simulink library "Lib_JARVISPH2_deVCU_Com"  (R2019b)
settings: Solver=ode45  StartTime=0.0  StopTime=10.0  RelTol=1e-3  EnableMultiTasking=on
settings Model: Creator=kmansour  LastModifiedBy=User
settings DataIOCC: LimitDataPoints=on  SaveFormat=Array  ReturnWorkspaceOutputs=off
settings OptimizationCC: LifeSpan=inf
settings DebuggingCC: AllowSymbolicDim=off  SFUnexpectedBacktrackingDiag=warning  SFNoUnconditionalDefaultTransitionDiag=warning  SFExecutionAtInitializationDiag=none  ArithmeticOperatorsInVariantConditions=warning
settings HardwareCC: ProdBitPerPointer=32  ProdBitPerSizeT=32  ProdBitPerPtrDiffT=32  ProdLargestAtomicFloat=None  ProdIntDivRoundTo=Undefined  ProdEndianess=Unspecified  ProdWordSize=32  ProdHWDeviceType=32-bit Generic
settings ModelReferenceCC: PropagateSignalLabelsOutOfModel=off
settings SFSimCC: SimUseLocalCustomCode=off  CustomCodeUndefinedFunction=UseInterfaceOnly
settings RTWCC: RTWUseLocalCustomCode=off
settings CodeAppCC: StateflowObjectComments=on
settings GRTTargetCC: TargetLangStandard=C89/C90 (ANSI)  GeneratePreprocessorConditionals=Disable all
settings ConfigComp: CovMetricSettings=dw  CovHtmlReporting=on  CovSaveCumulativeToWorkspaceVar=on  CovSaveSingleToWorkspaceVar=on  CovExternalEMLEnable=off

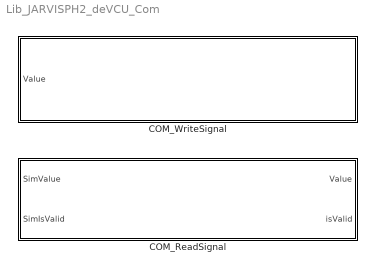
== system Lib_JARVISPH2_deVCU_Com ==
  COM_ReadSignal : Subsystem  TreatAsAtomicUnit=on  mask{PARAM_ID=APP_RX_ABS_EBS_AMBER_WARNING_LAMP_STATE}
      mask prompts: PARAM_ID "Choose Signal"
      mask TypeOptions PARAM_ID: APP_RX_ABS_EBS_AMBER_WARNING_LAMP_STATE | APP_RX_ABS_FULLY_OPERATIONAL | APP_RX_ABS_OFFROAD_SWITCH | APP_RX_ACCPEDAL_POS1 | APP_RX_ACC_PEDAL1LOWIDLESWITCH | APP_RX_ACC_PEDAL2KICKDOWNSWITCH | APP_RX_ACC_PEDAL_FAULT_BYTE1 | APP_RX_ACC_PEDAL_FAULT_BYTE2 | APP_RX_ACC_PEDAL_FAULT_BYTE3 | APP_RX_ACC_PEDAL_FAULT_BYTE4 | APP_RX_ACC_PEDAL_FAULT_BYTE5 | APP_RX_ACC_PEDAL_FAULT_BYTE6 | APP_RX_ACC_PEDAL_FAULT_BYTE7 | APP_RX_ACC_PEDAL_FAULT_BYTE8 | APP_RX_ACLTR_INTERLOCK_SWITCH | APP_RX_ACTUAL_TEMP_PUMP_AIRCOMP | APP_RX_AIR_COMPRESSOR_STATUS | APP_RX_AIR_SUSPENSION_SUPPLY_PRESSURE | APP_RX_AMBIENTTEMPERATURE | APP_RX_ANTI_LOCK_BRAKING_ABS_ACTIVE | APP_RX_ASR_BRAKE_CTRL_ACTIVE | APP_RX_ASR_ENG_CTRL_ACTIVE | APP_RX_ASR_HILL_HOLDER_SWITCH | APP_RX_ASR_OFFROAD_SWITCH | APP_RX_ATC_ASR_INFORMATION_SIGNAL | APP_RX_AUXILIARYVOLTAGE | APP_RX_AUXILIARYVOLTAGESTATUS | APP_RX_AUXILIARY_EQUIPMENT_SUPPLY_PRESS | APP_RX_BATTERY_SOH | APP_RX_BMS_CHECKSUM_126 | APP_RX_BMS_DCBUSVOLTAGE | APP_RX_BMS_HIGHESTINLETTEMP | APP_RX_BMS_HIGHESTOUTLETTEMP | APP_RX_BMS_MAXBATVOLTALLOWED | APP_RX_BMS_MAXCELLTEMP | APP_RX_BMS_MAXCONTCHRGCURRENT | APP_RX_BMS_MAXCONTDISCHRGCURRENT | APP_RX_BMS_MESSAGECOUNTER_126_HEARTBEAT | APP_RX_BMS_MINCELLTEMP | APP_RX_BMS_PACKCURRENT | APP_RX_BMS_PACKSTATE | APP_RX_BMS_PACKVOLTAGE | APP_RX_BMS_SOC | APP_RX_BMS_SUBPACK10STATUS | APP_RX_BMS_SUBPACK11STATUS | APP_RX_BMS_SUBPACK12STATUS | APP_RX_BMS_SUBPACK13STATUS | APP_RX_BMS_SUBPACK14STATUS | APP_RX_BMS_SUBPACK15STATUS | APP_RX_BMS_SUBPACK16STATUS | APP_RX_BMS_SUBPACK1STATUS | APP_RX_BMS_SUBPACK2STATUS | APP_RX_BMS_SUBPACK3STATUS | APP_RX_BMS_SUBPACK4STATUS | APP_RX_BMS_SUBPACK5STATUS | APP_RX_BMS_SUBPACK6STATUS | APP_RX_BMS_SUBPACK7STATUS | APP_RX_BMS_SUBPACK8STATUS | APP_RX_BMS_SUBPACK9STATUS | APP_RX_BMS_SYSTEMISORES | APP_RX_BMS_TMAX_CELL_ID | APP_RX_BMS_TMAX_SUBPACK_ID | APP_RX_BMS_TMIN_CELL_ID | APP_RX_BMS_TMIN_SUBPACK_ID | APP_RX_BRAKE_PEDAL_POSITION | APP_RX_CHECKSUM_122 | APP_RX_CHECKSUM_123 | APP_RX_COMMANDMODE_MCUCMD1RES | APP_RX_CONNECTED_STRING | APP_RX_DC_LINK_VOLTAGE_VCU_RX | APP_RX_DETECTED_STRING | APP_RX_EBS_BRAKE_SWITCH | APP_RX_EBS_RED_WARNING_LAMP_STATE | APP_RX_EM1_MESSAGECHECKSUM | APP_RX_EM1_MESSAGECOUNTER | APP_RX_EM1_OVR_CTRL_MODE_BRAKING | APP_RX_EM1_OVR_CTRL_MODE_DRIVING | APP_RX_EM1_OVR_CTRL_MODE_PRIO_BRAKING | APP_RX_EM1_OVR_CTRL_MODE_PRIO_DRIVING | APP_RX_EM1_REQ_TRQ_TRQ_LIMIT_BRAKING | APP_RX_EM1_REQ_TRQ_TRQ_LIMIT_DRIVING | APP_RX_EMERGENCYSTOP | APP_RX_EMITEMPERATURE | APP_RX_ENG_RET_SELECTION | APP_RX_EVENTID | APP_RX_FAULTDRIVECOVERWASOPENED | APP_RX_FAULTDRIVECOVERWASOPENEDSTATUS | APP_RX_FAULTINTERLOCKBATTERYCABLE | APP_RX_FAULTINTERLOCKBATTERYCABLESTATUS | APP_RX_FAULTINTERLOCKMOTORCABLE | APP_RX_FAULTINTERLOCKMOTORCABLESTATUS | APP_RX_FAULTPHASETOCHASSIS | APP_RX_FAULTPHASETOCHASSISSTATUS | APP_RX_FAULT_CODE_EHVS_VCU_RX | APP_RX_G1CHARGER_GUN_DETECTED | APP_RX_G1CHARGING_STATUS | APP_RX_G1DIFF_CURRENT_MEASURE | APP_RX_G1EVCC_READY | APP_RX_G1EVCC_STATUS_CODE | APP_RX_G1GUN_LOCK_FAULT | APP_RX_G1NEGATIVE_CONTACTOR_CONTROL | APP_RX_G1POSITIVE_CONTACTOR_CONTROL | APP_RX_G1TEMPERATURE1_FAULT | APP_RX_G1TEMPERATURE2_FAULT | APP_RX_G1TEMPERATURE_1_VAL | APP_RX_G1TEMPERATURE_2_VAL | APP_RX_G1VEHICLE_IMMOBILIZE | APP_RX_G1_GUNLOCKFEEDBACK | APP_RX_G2CHARGER_GUN_DETECTED | APP_RX_G2CHARGING_STATUS | APP_RX_G2DIFF_CURRENT_MEASURE | APP_RX_G2EVCC_READY | APP_RX_G2EVCC_STATUS_CODE | APP_RX_G2GUN_LOCK_FAULT | APP_RX_G2NEGATIVE_CONTACTOR_CONTROL | APP_RX_G2POSITIVE_CONTACTOR_CONTROL | APP_RX_G2TEMPERATURE1_FAULT | APP_RX_G2TEMPERATURE2_FAULT | APP_RX_G2TEMPERATURE_1_VAL | APP_RX_G2TEMPERATURE_2_VAL | APP_RX_G2VEHICLE_IMMOBILIZE | APP_RX_G2_GUNLOCKFEEDBACK | APP_RX_GEARSELECTOR_TESTSIG1 | APP_RX_GEARSELECTOR_TESTSIG2 | APP_RX_HALT_BRAKE_SWITCH | APP_RX_HIGHPOWERCURRENT | APP_RX_HIGHPOWERCURRENTSTATUS | APP_RX_HIGHPOWERVOLTAGE | APP_RX_HIGHPOWERVOLTAGESTATUS | APP_RX_HV_CONTACTOR_STATUS | APP_RX_MAXSAFEMOTORSPEEDFORWARD | APP_RX_MAXSAFEMOTORSPEEDFORWARDSTATUS | APP_RX_MAXSAFEMOTORSPEEDREVERSE | APP_RX_MAXSAFEMOTORSPEEDREVERSESTATUS | APP_RX_MCUPOLLINGVMU_BYTE1 | APP_RX_MCUPOLLINGVMU_BYTE2 | APP_RX_MCUPOLLINGVMU_BYTE3 | APP_RX_MCUPOLLINGVMU_BYTE4 | APP_RX_MCUPOLLINGVMU_BYTE5 | APP_RX_MCUPOLLINGVMU_BYTE6 | APP_RX_MCUPOLLINGVMU_BYTE7 | APP_RX_MCUPOLLINGVMU_BYTE8 | APP_RX_MCUTEMPERATURE | APP_RX_MCU_POLLING_MCU_BYTE1 | APP_RX_MCU_POLLING_MCU_BYTE2 | APP_RX_MCU_POLLING_MCU_BYTE3 | APP_RX_MCU_POLLING_MCU_BYTE4 | APP_RX_MCU_POLLING_MCU_BYTE5 | APP_RX_MCU_POLLING_MCU_BYTE6 | APP_RX_MCU_POLLING_MCU_BYTE7 | APP_RX_MCU_POLLING_MCU_BYTE8 | APP_RX_MESSAGECOUNTER_122 | APP_RX_MOTORANGLE | APP_RX_MOTORANGLESTATUS | APP_RX_MOTORSPEED | APP_RX_MOTORSPEEDSTATUS | APP_RX_MOTORTEMPERATURE | APP_RX_MOTORTORQUEESTIMATED | APP_RX_MOTORTORQUEESTIMATEDSTATUS | APP_RX_OPERATIONALMODE_MCUCMD1RES | APP_RX_OUTPUT_CURRENT_AIRCOMP | APP_RX_OUTPUT_CURRENT_EHVS | APP_RX_PARKING_AND_OR_TRAILER_AIR_PRESS | APP_RX_PNEUMATIC_SUPPLY_PRESSURE | APP_RX_PUMPCOMMUNICATIONFAULT | APP_RX_PUMPCURRENT | APP_RX_PUMPDRYRUNFAULT | APP_RX_PUMPFAULTLEVEL | APP_RX_PUMPOVERCURRENTFAULT | APP_RX_PUMPOVERVOLTAGEFAULT | APP_RX_PUMPSPEED | APP_RX_PUMPSTALLFAULT | APP_RX_PUMPTEMP | APP_RX_PUMPTHERMALFAULT | APP_RX_PUMPUNDERVOLTAGEFAULT | APP_RX_PUMPVOLTAGE | APP_RX_REGENDERATING | APP_RX_REGENDERATINGSTATUS | APP_RX_REGENTORQUEAVAIL | APP_RX_REGENTORQUEAVAILSTATUS | APP_RX_ROLLINGCOUNTER_MCUCMD1RESPONSE | APP_RX_ROLLINGCOUNTER_MCUCMD2RESPONSE | APP_RX_ROLLINGCOUNTER_MCUINFO1 | APP_RX_ROLLINGCOUNTER_MCUINFO2 | APP_RX_ROLLINGCOUNTER_MCUONEVENTINFO1 | APP_RX_ROLLINGCOUNTER_MCUTHERMAL2 | APP_RX_SA_OF_CTRLLINGDEVICEFORBRAKECTRL | APP_RX_SERVICE_BRAKE_CIRCUIT_1_AIR_PRES | APP_RX_SERVICE_BRAKE_CIRCUIT_2_AIR_PRES | APP_RX_SPEEDREDUCTIONREQUEST | APP_RX_STATEMCU | APP_RX_STATUSU0_FAULT_EHVS_VCU_RX | APP_RX_STATUSU0_OVERCURRENTFAULT_EHVS_V | APP_RX_STATUSU0_WARNING_EHVS_VCU_RX | APP_RX_STATUSU1_FAULT_AIRCOMP_VCU_RX | APP_RX_STATUSU1_OVERCURRENT_AIRCOMP_VCU | APP_RX_STATUSU1_OVERTEMP_AIRCOMP_VCU_RX | APP_RX_STATUSU1_WARNING_AIRCOMP_VCU_RX | APP_RX_SWITCHING_SYNC_STATUS | APP_RX_SYS_DTC | APP_RX_T2B_BMS_WORK_MODE | APP_RX_T2B_COMP_FREQUENCY | APP_RX_T2B_COOLANT_IN_TEMP | APP_RX_T2B_COOLANT_OUT_TEMP | APP_RX_T2B_FAULT_CODE | APP_RX_T2B_MODE | APP_RX_T2B_SIGNAL_LIFE | APP_RX_T2B_TMS_WORK_MODE | APP_RX_TRACTIONDERATING | APP_RX_TRACTIONDERATINGSTATUS | APP_RX_TRACTIONTORQUEAVAIL | APP_RX_TRACTIONTORQUEAVAILSTATUS | APP_RX_TRACTION_CTRL_OVR_SWITCH | APP_RX_TRAILER_ABS_STATUS | APP_RX_TRAILER_ABS_WARNING_SIGNAL | APP_RX_TRANSREQUEST_GEAR
      mask Display:
      | image(imread('devcu_final.png'),'top-left');
      | color('black');
      | port_label('input', 1, 'SimValue');
      | port_label('input', 2, 'SimIsValid');
      | port_label('output', 1, 'Value');
      | port_label('output', 2, 'isValid');
      | 
      | strCell =get_param(gcb, 'MaskValues');
      | strCell = strtrim(strCell);
      | str = strCell{1};
      | str = strrep(str, '_', '\_');
      | disp(str, 'texmode', 'on');
  COM_WriteSignal : Subsystem  TreatAsAtomicUnit=on  mask{PARAM_ID=APP_TX_ACKNOWLEDGEMENT}
      mask prompts: PARAM_ID "Choose Signal"
      mask TypeOptions PARAM_ID: APP_TX_ACKNOWLEDGEMENT | APP_TX_AIR_COMPRESSOR_AVAILABLE | APP_TX_AMBER_WARNING_LAMP_CHECK_HV | APP_TX_AP_LOW_IDLE_SWITCH | APP_TX_B2T_BATTERY_AVG_TEMP | APP_TX_B2T_BMS_WORK_MODE | APP_TX_B2T_COMP_SPEED_RESTRICTION | APP_TX_B2T_DIFFERENTIAL1 | APP_TX_B2T_DIFFERENTIAL2 | APP_TX_B2T_MODE | APP_TX_B2T_SET_TARGET_TEMP | APP_TX_B2T_SIGNAL_LIFE | APP_TX_B2T_TCELL_MAX | APP_TX_B2T_TCELL_MIN | APP_TX_B2T_TMS_CONTROL_CMD | APP_TX_BOOTNUMBER | APP_TX_CHECKSUM_200 | APP_TX_COMMANDMODEEXT | APP_TX_COMMANDMODE_VMUCMD2 | APP_TX_CONTROL0_EHPS | APP_TX_CONTROL1_AIRCOMP | APP_TX_DCDCONOFF | APP_TX_DISTANCE_TO_EMPTY_DTE | APP_TX_DTC_ACCHALLSENSOR_MALF_EXT_ERROR | APP_TX_DTC_ACCPDL_CHECKSUM_ERROR | APP_TX_DTC_ACCPDL_OUT_OF_CALIBRATION | APP_TX_DTC_ACCPDL_OVERTRAVEL_CLOCKWISE | APP_TX_DTC_ACCPDL_OVERTRAVEL_CNTRCW | APP_TX_DTC_ACC_HALLSENS_MALF_INT_ERROR | APP_TX_DTC_AIRCOMP_WARNING | APP_TX_DTC_AIR_COMPRESSOR_FAULT_ACTIVE | APP_TX_DTC_AIR_COMP_NOT_FUNCTIONAL | APP_TX_DTC_AUXBATT_UV_ACTIVE_WARN | APP_TX_DTC_AUX_BATTERY_OVER_VOLTAGE | APP_TX_DTC_AUX_BATTERY_UNDER_VOLTAGE | APP_TX_DTC_BATTERY_PACK_EMPTY_LOW_SOC | APP_TX_DTC_BATTTEMPLIMREACHEDDRNGCHRG | APP_TX_DTC_BATT_INTERNALLYWELDEDCONT | APP_TX_DTC_BRAKE_AIRCOMP_OVERCURRENT | APP_TX_DTC_BRAKE_AIRCOMP_OVERHEAT | APP_TX_DTC_CHARGE_COMPLETE | APP_TX_DTC_CHARSYSTEM_NOT_COMPATIBLE | APP_TX_DTC_DC_LINK_VOLTAGE_NOT_NORMAL | APP_TX_DTC_EHPS_FAULT_ACTIVE | APP_TX_DTC_EHPS_NOT_FUNCTIONAL | APP_TX_DTC_EHPS_OVERCURRENT | APP_TX_DTC_EHPS_WARNING | APP_TX_DTC_GUN1CHRG_CABLE_CHECK_FAILED | APP_TX_DTC_GUN1_CHARGING_AUTH_FAILED | APP_TX_DTC_GUN1_CHARGING_INIT_FAILED | APP_TX_DTC_GUN1_CONTACTORS_WELDED | APP_TX_DTC_GUN1_CONTACTOR_OPERFAULT | APP_TX_DTC_GUN1_LOCK_FAULT | APP_TX_DTC_GUN1_PRECHARGE_FAILED | APP_TX_DTC_GUN1_STOP_CHARGING_FLAG | APP_TX_DTC_GUN2_CHARGING_AUTH_FAILED | APP_TX_DTC_GUN2_CHARGING_INIT_FAILED | APP_TX_DTC_GUN2_CHRGCABLE_CHECK_FAILED | APP_TX_DTC_GUN2_CONTACTORS_WELDED | APP_TX_DTC_GUN2_CONT_OPERATION_FAULT | APP_TX_DTC_GUN2_LOCK_FAULT | APP_TX_DTC_GUN2_PRECHARGE_FAILED | APP_TX_DTC_GUN2_STOP_CHARGING_FLAG | APP_TX_DTC_HVAC_AMBIENT_SENSOR_FAULT | APP_TX_DTC_HVAC_CABIN_SENSOR_FAULT | APP_TX_DTC_HVAC_CAN_COMM_FAULT | APP_TX_DTC_HVAC_COMPRESSOR_FAULT | APP_TX_DTC_HVAC_COOLANT_LOW | APP_TX_DTC_HVAC_COOLANT_OVERHEAT | APP_TX_DTC_HVAC_DCDC_FAULT | APP_TX_DTC_HVAC_PRESSURE_FAULT | APP_TX_DTC_HVAC_PUMP_COMM_ERROR | APP_TX_DTC_HVAC_PUMP_DRY_RUN_FAULT | APP_TX_DTC_HVAC_PUMP_OVERCURRENT | APP_TX_DTC_HVAC_PUMP_OVERHEAT | APP_TX_DTC_HVAC_PUMP_STALL_FAULT | APP_TX_DTC_HVAC_SUCTION_TEMPSEN_FAULT | APP_TX_DTC_HVAC_WATERIN_SENSOR_FAULT | APP_TX_DTC_HVAC_WATEROUT_SENSOR_FAULT | APP_TX_DTC_HVIL_JB | APP_TX_DTC_IMBALANCED_STRING | APP_TX_DTC_IRREGULAR_INPUT_FROM_USER | APP_TX_DTC_KEY_NOT_DETECTED | APP_TX_DTC_LID_OPEN | APP_TX_DTC_LOSTCOMWITHMODULEINASTRING | APP_TX_DTC_LOST_COMM_WITH_HOST | APP_TX_DTC_LOST_COMM_WITH_SLAVES | APP_TX_DTC_MALFUNC_ACCPEDAL_WHILE_RUN | APP_TX_DTC_MANIPULATED_ACCPEDAL_VALUES | APP_TX_DTC_MCU_COMM_TIMEOUT_ERROR | APP_TX_DTC_MCU_EMERGENCY_STOP_REQUESTED | APP_TX_DTC_MCU_FAILED_TO_INITIALIZE | APP_TX_DTC_MCU_FAILURE | APP_TX_DTC_MCU_FAILUREDUETOOVERTEMP | APP_TX_DTC_MCU_FAULT_OBSERVED | APP_TX_DTC_MCU_OPERATIONAL_FAULT | APP_TX_DTC_MCU_OVERTEMP_WARNING | APP_TX_DTC_MCU_TEMP_LIMIT_REACHED | APP_TX_DTC_MOTOR_OVERTEMP_WARNING | APP_TX_DTC_MOTOR_TEMP_LIMIT_REACHED | APP_TX_DTC_PDU_CONTACTOR_WELDED | APP_TX_DTC_PDU_CONT_OPER_FAULT | APP_TX_DTC_PRECHARGE_FAULT | APP_TX_DTC_REFUSED_ENTER_NEUTRAL_MODE | APP_TX_DTC_REFUSED_ENTER_REVERSE_MODE | APP_TX_DTC_REFUSED_TO_ENTER_DRIVE_MODE | APP_TX_DTC_RISO_FAULT | APP_TX_DTC_SW_NOT_INSTALLED_PROPERLY | APP_TX_DTC_SYSTEM_CURRENT_CONTROL_FAULT | APP_TX_DTC_SYSTEM_LEVEL_BATTERY_FAULT | APP_TX_DTC_TCSCOOLANTINTEMPSENSOR_FAULT | APP_TX_DTC_TCSCOOLANTOUTTEMPSENS_FAULT | APP_TX_DTC_TCS_COOLANT_LEVEL_LOW | APP_TX_DTC_TCS_COOLANT_OUTLET_TEMP_HIGH | APP_TX_DTC_TCS_COOLANT_OVERHEAT | APP_TX_DTC_TCS_PUMP_COMM_FAULT | APP_TX_DTC_TCS_PUMP_OVERCURRENT_FAULT | APP_TX_DTC_TCS_PUMP_STALL_FAULT | APP_TX_DTC_TCS_PUMP_THERMAL_FAULT | APP_TX_DTC_TRQ_LIM_DUE_TO_MCU_DERATING | APP_TX_DTC_TRQ_LIM_DUE_TO_OVERCURRENT | APP_TX_DTC_TRQ_LIM_DUE_TO_OVERSPEED | APP_TX_DTC_TRQ_LIM_DUE_TO_THERMAL_LIM | APP_TX_DTC_TRQ_LIM_MCU_OUTOFORDER | APP_TX_DTC_VEHICLESYSTEM_NOT_COMPATIBLE | APP_TX_DTC_VEHICLE_CAN1_BUS_INACTIVE | APP_TX_DTC_VEHICLE_CAN2_BUS_INACTIVE | APP_TX_DTC_VEHICLE_CAN3_BUS_INACTIVE | APP_TX_EM1_ACTUAL_MAXAVAILRETPCTTRQ | APP_TX_EM1_ACTUAL_PCT_TORQUE | APP_TX_EM1_DRIVER_RETARDER_PCT_TORQUE | APP_TX_EM1_EMOTOR_OUTPUT_SHAFT_SPEED | APP_TX_EM1_ER_SEQUENCE_NUMBER | APP_TX_EM1_REF_ENG_TORQ | APP_TX_EM1_REF_RET_TORQ | APP_TX_EM1_RET_LOCATION | APP_TX_EM1_RET_SELECTION_NON_ENG | APP_TX_EM1_RET_TYPE | APP_TX_EM1_SA_OF_CTRL_DEVICE | APP_TX_EM1_TORQUE_MODE_DRIVING_BRAKING | APP_TX_G1BATTERY_PACK_PRESENT_VOLT | APP_TX_G1CHARG_COMP_FLAG | APP_TX_G1EV_CONTI_CHARG_CUR_LIMIT | APP_TX_G1EV_ERROR_CODE | APP_TX_G1EV_MAX_CHARG_CUR_LIMIT | APP_TX_G1EV_READY_FLAG | APP_TX_G1NOMI_BATT_CAPA | APP_TX_G1REMAIN_BATT_CAPA | APP_TX_G1SOC | APP_TX_G1VEHI_STOP_CHARG_FLAG | APP_TX_G2BATTERY_PACK_PRESENT_VOLT | APP_TX_G2CHARG_COMP_FLAG | APP_TX_G2EV_CONTI_CHARG_CUR_LIMIT | APP_TX_G2EV_ERROR_CODE | APP_TX_G2EV_MAX_CHARG_CUR_LIMIT | APP_TX_G2EV_READY_FLAG | APP_TX_G2NOMI_BATT_CAPA | APP_TX_G2REMAIN_BATT_CAPA | APP_TX_G2SOC | APP_TX_G2VEHI_STOP_CHARG_FLAG | APP_TX_HIGH_VOLT_BATT_1_FAULT | APP_TX_HIGH_VOLT_BATT_2_FAULT | APP_TX_HOST_BMSSTATEREQUEST | APP_TX_HV_READY | APP_TX_HV_SYSTEM_VOLTAGE | APP_TX_INVERTER_TEMPERATURE | APP_TX_MAJORMCUPROTOCOL | APP_TX_MAXBATTERYVOLTAGE | APP_TX_MAXBATTERYVOLTAGESTATUS | APP_TX_MAXCHARGECURRENT | APP_TX_MAXCHARGECURRENTSTATUS | APP_TX_MAXDISCHARGECURRENT | APP_TX_MAXDISCHARGECURRENTSTATUS | APP_TX_MCUREQUESTID | APP_TX_MESSAGECOUNTER_200 | APP_TX_MINBATTERYVOLTAGE | APP_TX_MINBATTERYVOLTAGESTATUS | APP_TX_MINORMCUPROTOCOL | APP_TX_MOTOR_INVERTER_OVER_TEMP_WARNING | APP_TX_MOTOR_SPEED | APP_TX_NOMINAL_FRICTION_PCT_TORQ | APP_TX_OPERATIONALMODE | APP_TX_OPERATIONREQUEST_VMUCMD1 | APP_TX_PARKING_BRAKE_SWITCH | APP_TX_REBOOT_REQUEST | APP_TX_RED_STOP_LAMP_STOP_HV | APP_TX_REFERENCECOMMANDMODE | APP_TX_REFERENCESPEEDCOMMAND | APP_TX_REFERENCETORQUECOMMAND | APP_TX_REGEN_BRAKING_AVAILABLE | APP_TX_ROAD_SPEED_LIMIT_STATUS | APP_TX_ROLLINGCOUNTER_VMUCMD1 | APP_TX_ROLLINGCOUNTER_VMUCMD2 | APP_TX_ROLLINGCOUNTER_VMUCMDSAFETY | APP_TX_SPEEDCOMMAND | APP_TX_SPEEDCOMMANDSTATUS | APP_TX_TARGETVALUE | APP_TX_TORQUECOMMAND | APP_TX_TORQUECOMMANDSTATUS | APP_TX_TPCM_EM1_BAM | APP_TX_TPCM_EM1_BYT | APP_TX_TPCM_EM1_PGN | APP_TX_TPCM_TPDT_5THFRAME | APP_TX_TPCM_TPDT_FRAMES | APP_TX_TRACTION_BATTERY_CURRENT | APP_TX_TRACTION_BATTERY_SOC | APP_TX_TRACTION_BATTERY_SOH | APP_TX_TRACTION_BATTERY_TEMPERATURE | APP_TX_TRACTION_BATT_CONNECTED | APP_TX_TRACT_BATT_OVER_TEMPE_WAR | APP_TX_TRAC_SYSTEM_REDUCED_PER_MODE | APP_TX_TRANSM_READY_FOR_BRAKE_RELEASE | APP_TX_TRAS_CURRENT_RANGE | APP_TX_VCU_PARALOGCOOLENTIN | APP_TX_VCU_PARALOGCOOLENTOUT | APP_TX_VCU_PARALOG_ACCPEDAL | APP_TX_VCU_PARALOG_MOTORRPM | APP_TX_VCU_PARALOG_TRQCMD | APP_TX_VCU_PARALOG_VEHSPEED | APP_TX_VEHICLE_PLUGGED_IN | APP_TX_VEHICLE_SPEED | APP_TX_VMUREQUESTID | APP_TX_WHEEL_BASED_VEHICLE_SPEED
      mask Display:
      | image(imread('devcu_final.png'),'top-right');
      | color('black');
      | port_label('input', 1, 'Value');
      | 
      | strCell =get_param(gcb, 'MaskValues');
      | strCell = strtrim(strCell);
      | str = strCell{1};
      | str = strrep(str, '_', '\_');
      | disp(str, 'texmode', 'on');

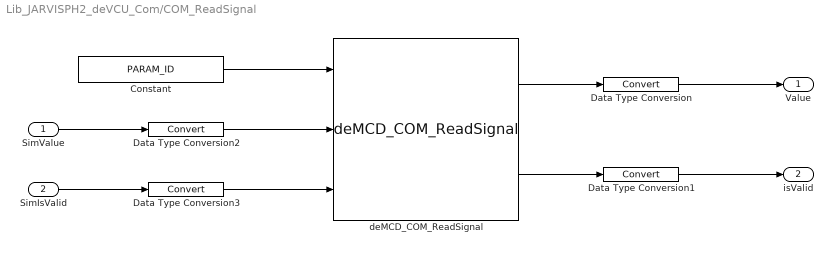
== system Lib_JARVISPH2_deVCU_Com/COM_ReadSignal ==
  SimValue : Inport
  SimIsValid : Inport  Port=2
  Constant : Constant  Value=PARAM_ID
  Data Type Conversion{,1..3} (4 alike) : DataTypeConversion
  deMCD_COM_ReadSignal : S-Function  FunctionName=deMCD_COM_ReadSignal  SFunctionDeploymentMode=off  EnableBusSupport=off
      mask Display:
      | image(imread('logo_deMCD_white_background.png'),'center');
      | color('black');
      | port_label('input', 1, 'ID');
      | port_label('input', 2, 'SimValue');
      | port_label('input', 3, 'SimIsValid');
      | port_label('output', 1, 'Value');
      | port_label('output', 2, 'isValid');
  Value : Outport
  isValid : Outport  Port=2
  wires:
  Constant/1 -> deMCD_COM_ReadSignal/1
  deMCD_COM_ReadSignal/1 -> Data Type Conversion/1
  deMCD_COM_ReadSignal/2 -> Data Type Conversion1/1
  Data Type Conversion/1 -> Value/1
  Data Type Conversion1/1 -> isValid/1
  SimValue/1 -> Data Type Conversion2/1
  Data Type Conversion2/1 -> deMCD_COM_ReadSignal/2
  Data Type Conversion3/1 -> deMCD_COM_ReadSignal/3
  SimIsValid/1 -> Data Type Conversion3/1

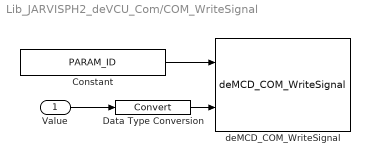
== system Lib_JARVISPH2_deVCU_Com/COM_WriteSignal ==
  Value : Inport
  Constant : Constant  Value=PARAM_ID
  Data Type Conversion : DataTypeConversion
  deMCD_COM_WriteSignal : S-Function  FunctionName=deMCD_COM_WriteSignal  SFunctionDeploymentMode=off  EnableBusSupport=off
      mask Display:
      | image(imread('logo_deMCD_white_background.png'),'center');
      | color('black');
      | port_label('input', 1, 'ID');
      | port_label('input', 2, 'Value');
  wires:
  Value/1 -> Data Type Conversion/1
  Constant/1 -> deMCD_COM_WriteSignal/1
  Data Type Conversion/1 -> deMCD_COM_WriteSignal/2
